simulink model "Dpcm"  (R2021a)
settings: Solver=VariableStepAuto  StartTime=0.0  StopTime=10.0  RelTol=1e-3
libraries: dspquant2 x2, dsparch4 x1, dspsigops x1
settings Model: Creator=GUNA  LastModifiedBy=GUNA

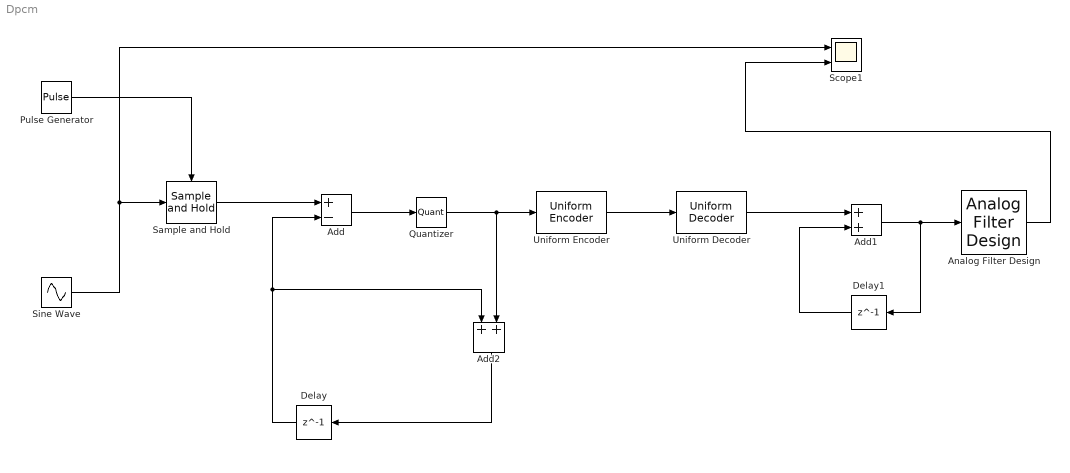
== system Dpcm ==
  Add : Sum  Inputs=+-
  Add1 : Sum
  Add2 : Sum
  Analog Filter Design : dsparch4/Analog Filter Design  method=Butterworth  filttype=Lowpass  N=16  Wlo=2*pi*40  Whi=80  Rp=2  Rs=40
  Delay : Delay  DelayLength=1  InitialCondition=0
  Delay1 : Delay  DelayLength=1  InitialCondition=0
  Pulse Generator : DiscretePulseGenerator  PulseType=Time based  Period=1/400  PulseWidth=5
  Quantizer : Quantizer  QuantizationInterval=0.1
  Sample and Hold : dspsigops/Sample and Hold  trig=Rising edge  initCond=0  latchinput=off
  Scope1 : Scope  NumInputPorts=2
  Sine Wave : Sin  Frequency=2*pi*20  SampleTime=0
  Uniform Decoder : dspquant2/Uniform Decoder  peak=3  bits=16  overflowMode=Saturate  otype=Double
      settings: SourceProductBaseCode=DS
  Uniform Encoder : dspquant2/Uniform Encoder  peak=3  bits=16  otype=Unsigned integer
  wires:
  Pulse Generator/1 -> Sample and Hold/Trigger
  Sine Wave/1 -> Scope1/1, Sample and Hold/1
  Sample and Hold/1 -> Add/1
  Add1/1 -> Delay1/1, Analog Filter Design/1
  Add/1 -> Quantizer/1
  Quantizer/1 -> Uniform Encoder/1, Add2/2
  Add2/1 -> Delay/1
  Delay/1 -> Add2/1, Add/2
  Uniform Encoder/1 -> Uniform Decoder/1
  Uniform Decoder/1 -> Add1/1
  Delay1/1 -> Add1/2
  Analog Filter Design/1 -> Scope1/2
